simulink model "PFC_69C_03_06_V01_3Phase_3_2KW"  (R2022b)
settings: Solver=FixedStepAuto  StartTime=0.0  StopTime=Inf  RelTol=1e-3  EnableMultiTasking=on
model workspace (MAT data in the model file):
  ADC_Gain = 1241.21212121
  DAC_Gain = 0.000805860805861
  Inductor_Current_Divider_Gain_Phase_A = 33.4
  Inductor_Current_Divider_Gain_Phase_B = 33.4
  Vbulk_Divider_Gain = 276.854928018
  Vin_Divider_Gain = 556.17352614
undefined symbols (not defined in the file or in its folder): GPTRIP1SEL, GPTRIP2SEL, SCI_A_Transmit, SCI_A_Transmit_Current_Suffix, SCI_A_Transmit_one_shot_Suffix, SCI_A_Transmit_Polarity_Suffix, SCI_A_Transmit_relay_Suffix, SCI_A_Transmit_Vbulk_Suffix, SCI_A_Transmit_Vin_rms_Suffix, SCI_A_Transmit_Vin_Suffix, SCI_A_Transmit_Vmid_Suffix, SCI_A_Transmit_Vp_Suffix, SCI_A_Transmit_Vpfc_Suffix, TZ1, TZ2
libraries: c280xlib x38, c2802xlib x34, simulink x17, c2000lib x1
(part 1 of 8)
settings Model: ExtModeTrigDuration=8  Creator=natchammaimuthu  LastModifiedBy=natchammaimuthu
settings OptimizationCC: DefaultUnderspecifiedDataType=single  EnhancedBackFolding=on  PassReuseOutputArgsAs=Individual arguments  MaxStackSize=1024  OptimizeBlockOrder=speed  DifferentSizesBufferReuse=on  OptimizationCustomize=off  DenormalBehavior=FlushToZero  EfficientTunableParamExpr=on
settings DebuggingCC: MultiTaskDSMMsg=none  ParameterPrecisionLossMsg=none  ParameterTunabilityLossMsg=error
settings HardwareCC: ProdBitPerChar=16  ProdBitPerInt=16  ProdBitPerPointer=32  ProdBitPerSizeT=32  ProdBitPerPtrDiffT=32  ProdLargestAtomicInteger=Integer  ProdLargestAtomicFloat=None  ProdWordSize=16  ProdLongLongMode=on  ProdHWDeviceType=Texas Instruments->C2000
settings SFSimCC: MATLABDynamicMemAlloc=off
settings RTWCC: Description=Embedded Coder  SystemTargetFile=ert.tlc  HardwareBoard=TI Piccolo F2806x  TLCOptions=-aInlineSetEventsForThisBaseRateFcn=TLC_FALSE -aSuppressMultiTaskScheduler=TLC_FALSE -aRateBasedStepFcn=1  TemplateMakefile=ert_default_tmf  Toolchain=Texas Instruments Code Composer Studio (C2000)
settings CodeAppCC: ForceParamTrailComments=on  IgnoreCustomStorageClasses=off  OperatorAnnotations=on  SimulinkDataObjDesc=on  SFDataObjDesc=on  InsertBlockDesc=on
settings ERTTargetCC: CodeReplacementLibrary=TI C28x  ExtModeTransport=4  ExtModeStaticAlloc=on  ExtModeAutomaticAllocSize=off  ExtModeMexFile=ext_xcp  ExtModeIntrfLevel=Level2 - Open

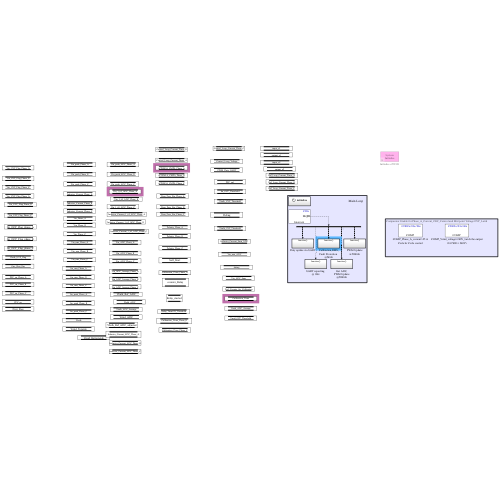
[thumbnail: Simulink's stored preview of the top-level diagram]
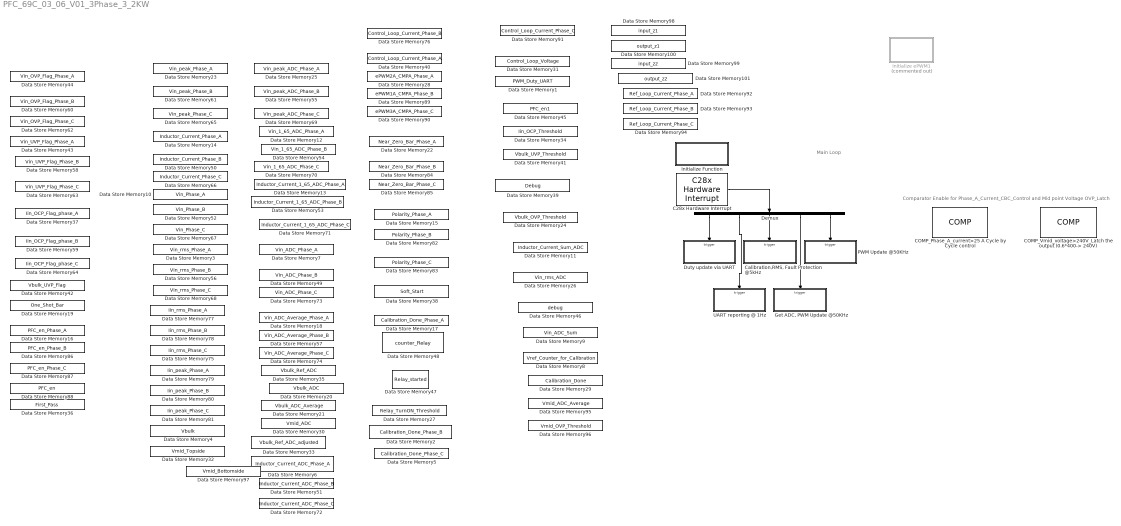
== system PFC_69C_03_06_V01_3Phase_3_2KW ==
  note: Comparator Enable for Phase_A_Current_CBC_Control and Mid point Voltage OVP_Latch
  note: Main Loop
  C28x Hardware Interrupt : c2000lib/Scheduling/C28x Hardware Interrupt  irqnumbers=[9 3 3 3 1]  pienumbers=[1 7 4 2 1]  irqpriorities=[10 9 8 7 6]  irqpreempts=[1 1 1 0 0]  showinput=off  dspchiptype=C280X
  COMP_Phase_A_current>25 A Cycle by Cycle control : c2802xlib/COMP  comparatorModule=Comparator 1  comparatorGPIO1=[]  comparatorGPIO2=0  comparatorSource=Internal DAC  DACOutputValue=744  inverterCircuit=off  synchronizationSelect=Asynchronous  qualificationPeriod=Passed through  Ts=-1
      settings: LibrarySourceBlock=c2806xlib/COMP
  COMP_Vmid_voltage>240V_Latch the output (0.6*400-> 240V) : c2802xlib/COMP  comparatorModule=Comparator 2  comparatorGPIO1=[]  comparatorGPIO2=0  comparatorSource=Internal DAC  DACOutputValue=479  inverterCircuit=off  synchronizationSelect=Asynchronous  qualificationPeriod=Passed through  Ts=-1
      settings: LibrarySourceBlock=c2806xlib/COMP
  "Calibration,RMS, Fault Protection @5kHz" : Subsystem  TreatAsAtomicUnit=on
  Data Store Memory1 : DataStoreMemory  DataStoreName=PWM_Duty_UART  WriteAfterWriteMsg=warning  InitialValue=5  ShowAdditionalParam=off  OutDataTypeStr=double
  Data Store Memory10 : DataStoreMemory  DataStoreName=Vin_Phase_A  WriteAfterWriteMsg=warning  ShowAdditionalParam=off  OutDataTypeStr=double
  Data Store Memory100 : DataStoreMemory  DataStoreName=output_z1  WriteAfterWriteMsg=warning  ShowAdditionalParam=off  OutDataTypeStr=double
  Data Store Memory101 : DataStoreMemory  DataStoreName=output_z2  WriteAfterWriteMsg=warning  ShowAdditionalParam=off  OutDataTypeStr=double
  Data Store Memory11 : DataStoreMemory  DataStoreName=Inductor_Current_Sum_ADC  WriteAfterWriteMsg=warning  ShowAdditionalParam=off  OutDataTypeStr=double
  Data Store Memory12 : DataStoreMemory  DataStoreName=Vin_1_65_ADC_Phase_A  WriteAfterWriteMsg=warning  ShowAdditionalParam=off  OutDataTypeStr=double
  Data Store Memory13 : DataStoreMemory  DataStoreName=Inductor_Current_1_65_ADC_Phase_A  WriteAfterWriteMsg=warning  ShowAdditionalParam=off  OutDataTypeStr=double
  Data Store Memory14 : DataStoreMemory  DataStoreName=Inductor_Current_Phase_A  WriteAfterWriteMsg=warning  ShowAdditionalParam=off  OutDataTypeStr=double
  Data Store Memory15 : DataStoreMemory  DataStoreName=Polarity_Phase_A  WriteAfterWriteMsg=warning  InitialValue=10  ShowAdditionalParam=off
  Data Store Memory16 : DataStoreMemory  DataStoreName=PFC_en_Phase_A  WriteAfterWriteMsg=warning  ShowAdditionalParam=off
  Data Store Memory17 : DataStoreMemory  DataStoreName=Calibration_Done_Phase_A  WriteAfterWriteMsg=warning  ShowAdditionalParam=off  OutDataTypeStr=double
  Data Store Memory18 : DataStoreMemory  DataStoreName=Vin_ADC_Average_Phase_A  WriteAfterWriteMsg=warning  ShowAdditionalParam=off
  Data Store Memory19 : DataStoreMemory  DataStoreName=One_Shot_Bar  WriteAfterWriteMsg=warning  InitialValue=1  ShowAdditionalParam=off  OutDataTypeStr=double
  Data Store Memory2 : DataStoreMemory  DataStoreName=Calibration_Done_Phase_B  WriteAfterWriteMsg=warning  ShowAdditionalParam=off  OutDataTypeStr=double
  Data Store Memory20 : DataStoreMemory  DataStoreName=Vbulk_ADC  WriteAfterWriteMsg=warning  ShowAdditionalParam=off
  Data Store Memory21 : DataStoreMemory  DataStoreName=Vbulk_ADC_Average  WriteAfterWriteMsg=warning  ShowAdditionalParam=off
  Data Store Memory22 : DataStoreMemory  DataStoreName=Near_Zero_Bar_Phase_A  WriteAfterWriteMsg=warning  InitialValue=10  ShowAdditionalParam=off
  Data Store Memory23 : DataStoreMemory  DataStoreName=Vin_peak_Phase_A  WriteAfterWriteMsg=warning  ShowAdditionalParam=off  OutDataTypeStr=double
  Data Store Memory24 : DataStoreMemory  DataStoreName=Vbulk_OVP_Threshold  WriteAfterWriteMsg=warning  InitialValue=100  ShowAdditionalParam=off
  Data Store Memory25 : DataStoreMemory  DataStoreName=Vin_peak_ADC_Phase_A  WriteAfterWriteMsg=warning  ShowAdditionalParam=off  OutDataTypeStr=double
  Data Store Memory26 : DataStoreMemory  DataStoreName=Vin_rms_ADC  WriteAfterWriteMsg=warning  InitialValue=10  ShowAdditionalParam=off
  Data Store Memory27 : DataStoreMemory  DataStoreName=Relay_TurnON_Threshold  WriteAfterWriteMsg=warning  InitialValue=10  ShowAdditionalParam=off
  Data Store Memory28 : DataStoreMemory  DataStoreName=ePWM2A_CMPA_Phase_A  WriteAfterWriteMsg=warning  ShowAdditionalParam=off
  Data Store Memory29 : DataStoreMemory  DataStoreName=Calibration_Done  WriteAfterWriteMsg=warning  ShowAdditionalParam=off  OutDataTypeStr=double
  Data Store Memory3 : DataStoreMemory  DataStoreName=Vin_rms_Phase_A  WriteAfterWriteMsg=warning  InitialValue=10  ShowAdditionalParam=off
  Data Store Memory30 : DataStoreMemory  DataStoreName=Vmid_ADC  WriteAfterWriteMsg=warning  InitialValue=10  ShowAdditionalParam=off  OutDataTypeStr=double
  Data Store Memory31 : DataStoreMemory  DataStoreName=Control_Loop_Voltage  WriteAfterWriteMsg=warning  InitialValue=100  ShowAdditionalParam=off
  Data Store Memory32 : DataStoreMemory  DataStoreName=Vmid_Topside  WriteAfterWriteMsg=warning  InitialValue=10  ShowAdditionalParam=off  OutDataTypeStr=double
  Data Store Memory33 : DataStoreMemory  DataStoreName=Vbulk_Ref_ADC_adjusted  WriteAfterWriteMsg=warning  InitialValue=10  ShowAdditionalParam=off  OutDataTypeStr=double
  Data Store Memory34 : DataStoreMemory  DataStoreName=Iin_OCP_Threshold  WriteAfterWriteMsg=warning  ShowAdditionalParam=off  OutDataTypeStr=double
  Data Store Memory35 : DataStoreMemory  DataStoreName=Vbulk_Ref_ADC  WriteAfterWriteMsg=warning  InitialValue=10  ShowAdditionalParam=off  OutDataTypeStr=double
  Data Store Memory36 : DataStoreMemory  DataStoreName=First_Pass  WriteAfterWriteMsg=warning  ShowAdditionalParam=off  OutDataTypeStr=double
  Data Store Memory37 : DataStoreMemory  DataStoreName=Iin_OCP_Flag_phase_A  WriteAfterWriteMsg=warning  InitialValue=1  ShowAdditionalParam=off  OutDataTypeStr=double
  Data Store Memory38 : DataStoreMemory  DataStoreName=Soft_Start  WriteAfterWriteMsg=warning  InitialValue=10  ShowAdditionalParam=off  OutDataTypeStr=double
  Data Store Memory39 : DataStoreMemory  DataStoreName=Debug  WriteAfterWriteMsg=warning  InitialValue=10  ShowAdditionalParam=off  OutDataTypeStr=double
  Data Store Memory4 : DataStoreMemory  DataStoreName=Vbulk  WriteAfterWriteMsg=warning  ShowAdditionalParam=off  OutDataTypeStr=double
  Data Store Memory40 : DataStoreMemory  DataStoreName=Control_Loop_Current_Phase_A  WriteAfterWriteMsg=warning  InitialValue=100  ShowAdditionalParam=off
  Data Store Memory41 : DataStoreMemory  DataStoreName=Vbulk_UVP_Threshold  WriteAfterWriteMsg=warning  InitialValue=-10  VectorParams1D=off  ShowAdditionalParam=off  OutDataTypeStr=double
  Data Store Memory42 : DataStoreMemory  DataStoreName=Vbulk_UVP_Flag  WriteAfterWriteMsg=warning  ShowAdditionalParam=off
  Data Store Memory43 : DataStoreMemory  DataStoreName=Vin_UVP_Flag_Phase_A  WriteAfterWriteMsg=warning  ShowAdditionalParam=off
  Data Store Memory44 : DataStoreMemory  DataStoreName=Vin_OVP_Flag_Phase_A  WriteAfterWriteMsg=warning  ShowAdditionalParam=off
  Data Store Memory45 : DataStoreMemory  DataStoreName=PFC_en1  WriteAfterWriteMsg=warning  ShowAdditionalParam=off
  Data Store Memory46 : DataStoreMemory  DataStoreName=debug  WriteAfterWriteMsg=warning  ShowAdditionalParam=off
  Data Store Memory47 : DataStoreMemory  DataStoreName=Relay_started  WriteAfterWriteMsg=warning  ShowAdditionalParam=off
  Data Store Memory48 : DataStoreMemory  DataStoreName=counter_Relay  WriteAfterWriteMsg=warning  ShowAdditionalParam=off
  Data Store Memory49 : DataStoreMemory  DataStoreName=Vin_ADC_Phase_B  WriteAfterWriteMsg=warning  ShowAdditionalParam=off
  Data Store Memory5 : DataStoreMemory  DataStoreName=Calibration_Done_Phase_C  WriteAfterWriteMsg=warning  ShowAdditionalParam=off  OutDataTypeStr=double
  Data Store Memory50 : DataStoreMemory  DataStoreName=Inductor_Current_Phase_B  WriteAfterWriteMsg=warning  ShowAdditionalParam=off  OutDataTypeStr=double
  Data Store Memory51 : DataStoreMemory  DataStoreName=Inductor_Current_ADC_Phase_B  WriteAfterWriteMsg=warning  ShowAdditionalParam=off  OutDataTypeStr=double
  Data Store Memory52 : DataStoreMemory  DataStoreName=Vin_Phase_B  WriteAfterWriteMsg=warning  ShowAdditionalParam=off  OutDataTypeStr=double
  Data Store Memory53 : DataStoreMemory  DataStoreName=Inductor_Current_1_65_ADC_Phase_B  WriteAfterWriteMsg=warning  ShowAdditionalParam=off  OutDataTypeStr=double
  Data Store Memory54 : DataStoreMemory  DataStoreName=Vin_1_65_ADC_Phase_B  WriteAfterWriteMsg=warning  ShowAdditionalParam=off  OutDataTypeStr=double
  Data Store Memory55 : DataStoreMemory  DataStoreName=Vin_peak_ADC_Phase_B  WriteAfterWriteMsg=warning  ShowAdditionalParam=off  OutDataTypeStr=double
  Data Store Memory56 : DataStoreMemory  DataStoreName=Vin_rms_Phase_B  WriteAfterWriteMsg=warning  InitialValue=10  ShowAdditionalParam=off
  Data Store Memory57 : DataStoreMemory  DataStoreName=Vin_ADC_Average_Phase_B  WriteAfterWriteMsg=warning  ShowAdditionalParam=off
  Data Store Memory58 : DataStoreMemory  DataStoreName=Vin_UVP_Flag_Phase_B  WriteAfterWriteMsg=warning  ShowAdditionalParam=off
  Data Store Memory59 : DataStoreMemory  DataStoreName=Iin_OCP_Flag_phase_B  WriteAfterWriteMsg=warning  InitialValue=1  ShowAdditionalParam=off  OutDataTypeStr=double
  Data Store Memory6 : DataStoreMemory  DataStoreName=Inductor_Current_ADC_Phase_A  WriteAfterWriteMsg=warning  ShowAdditionalParam=off  OutDataTypeStr=double
  Data Store Memory60 : DataStoreMemory  DataStoreName=Vin_OVP_Flag_Phase_B  WriteAfterWriteMsg=warning  ShowAdditionalParam=off
  Data Store Memory61 : DataStoreMemory  DataStoreName=Vin_peak_Phase_B  WriteAfterWriteMsg=warning  ShowAdditionalParam=off  OutDataTypeStr=double
  Data Store Memory62 : DataStoreMemory  DataStoreName=Vin_OVP_Flag_Phase_C  WriteAfterWriteMsg=warning  ShowAdditionalParam=off
  Data Store Memory63 : DataStoreMemory  DataStoreName=Vin_UVP_Flag_Phase_C  WriteAfterWriteMsg=warning  ShowAdditionalParam=off
  Data Store Memory64 : DataStoreMemory  DataStoreName=Iin_OCP_Flag_phase_C  WriteAfterWriteMsg=warning  InitialValue=1  ShowAdditionalParam=off  OutDataTypeStr=double
  Data Store Memory65 : DataStoreMemory  DataStoreName=Vin_peak_Phase_C  WriteAfterWriteMsg=warning  ShowAdditionalParam=off  OutDataTypeStr=double
  Data Store Memory66 : DataStoreMemory  DataStoreName=Inductor_Current_Phase_C  WriteAfterWriteMsg=warning  ShowAdditionalParam=off  OutDataTypeStr=double
  Data Store Memory67 : DataStoreMemory  DataStoreName=Vin_Phase_C  WriteAfterWriteMsg=warning  ShowAdditionalParam=off  OutDataTypeStr=double
  Data Store Memory68 : DataStoreMemory  DataStoreName=Vin_rms_Phase_C  WriteAfterWriteMsg=warning  InitialValue=10  ShowAdditionalParam=off
  Data Store Memory69 : DataStoreMemory  DataStoreName=Vin_peak_ADC_Phase_C  WriteAfterWriteMsg=warning  ShowAdditionalParam=off  OutDataTypeStr=double
  Data Store Memory7 : DataStoreMemory  DataStoreName=Vin_ADC_Phase_A  WriteAfterWriteMsg=warning  ShowAdditionalParam=off
  Data Store Memory70 : DataStoreMemory  DataStoreName=Vin_1_65_ADC_Phase_C  WriteAfterWriteMsg=warning  ShowAdditionalParam=off  OutDataTypeStr=double
  Data Store Memory71 : DataStoreMemory  DataStoreName=Inductor_Current_1_65_ADC_Phase_C  WriteAfterWriteMsg=warning  ShowAdditionalParam=off  OutDataTypeStr=double
  Data Store Memory72 : DataStoreMemory  DataStoreName=Inductor_Current_ADC_Phase_C  WriteAfterWriteMsg=warning  ShowAdditionalParam=off  OutDataTypeStr=double
  Data Store Memory73 : DataStoreMemory  DataStoreName=Vin_ADC_Phase_C  WriteAfterWriteMsg=warning  ShowAdditionalParam=off
  Data Store Memory74 : DataStoreMemory  DataStoreName=Vin_ADC_Average_Phase_C  WriteAfterWriteMsg=warning  ShowAdditionalParam=off
  Data Store Memory75 : DataStoreMemory  DataStoreName=Iin_rms_Phase_C  WriteAfterWriteMsg=warning  InitialValue=10  ShowAdditionalParam=off
  Data Store Memory76 : DataStoreMemory  DataStoreName=Control_Loop_Current_Phase_B  WriteAfterWriteMsg=warning  InitialValue=100  ShowAdditionalParam=off
  Data Store Memory77 : DataStoreMemory  DataStoreName=Iin_rms_Phase_A  WriteAfterWriteMsg=warning  InitialValue=10  ShowAdditionalParam=off
  Data Store Memory78 : DataStoreMemory  DataStoreName=Iin_rms_Phase_B  WriteAfterWriteMsg=warning  InitialValue=10  ShowAdditionalParam=off
  Data Store Memory79 : DataStoreMemory  DataStoreName=Iin_peak_Phase_A  WriteAfterWriteMsg=warning  ShowAdditionalParam=off  OutDataTypeStr=double
  Data Store Memory8 : DataStoreMemory  DataStoreName=Vref_Counter_for_Calibration  WriteAfterWriteMsg=warning  ShowAdditionalParam=off
  Data Store Memory80 : DataStoreMemory  DataStoreName=Iin_peak_Phase_B  WriteAfterWriteMsg=warning  ShowAdditionalParam=off  OutDataTypeStr=double
  Data Store Memory81 : DataStoreMemory  DataStoreName=Iin_peak_Phase_C  WriteAfterWriteMsg=warning  ShowAdditionalParam=off  OutDataTypeStr=double
  Data Store Memory82 : DataStoreMemory  DataStoreName=Polarity_Phase_B  WriteAfterWriteMsg=warning  InitialValue=10  ShowAdditionalParam=off
  Data Store Memory83 : DataStoreMemory  DataStoreName=Polarity_Phase_C  WriteAfterWriteMsg=warning  InitialValue=10  ShowAdditionalParam=off
  Data Store Memory84 : DataStoreMemory  DataStoreName=Near_Zero_Bar_Phase_B  WriteAfterWriteMsg=warning  InitialValue=10  ShowAdditionalParam=off
  Data Store Memory85 : DataStoreMemory  DataStoreName=Near_Zero_Bar_Phase_C  WriteAfterWriteMsg=warning  InitialValue=10  ShowAdditionalParam=off
  Data Store Memory86 : DataStoreMemory  DataStoreName=PFC_en_Phase_B  WriteAfterWriteMsg=warning  ShowAdditionalParam=off
  Data Store Memory87 : DataStoreMemory  DataStoreName=PFC_en_Phase_C  WriteAfterWriteMsg=warning  ShowAdditionalParam=off
  Data Store Memory88 : DataStoreMemory  DataStoreName=PFC_en  WriteAfterWriteMsg=warning  ShowAdditionalParam=off
  Data Store Memory89 : DataStoreMemory  DataStoreName=ePWM1A_CMPA_Phase_B  WriteAfterWriteMsg=warning  ShowAdditionalParam=off
  Data Store Memory9 : DataStoreMemory  DataStoreName=Vin_ADC_Sum  WriteAfterWriteMsg=warning  ShowAdditionalParam=off  OutDataTypeStr=double
  Data Store Memory90 : DataStoreMemory  DataStoreName=ePWM3A_CMPA_Phase_C  WriteAfterWriteMsg=warning  ShowAdditionalParam=off
  Data Store Memory91 : DataStoreMemory  DataStoreName=Control_Loop_Current_Phase_C  WriteAfterWriteMsg=warning  InitialValue=100  ShowAdditionalParam=off
  Data Store Memory92 : DataStoreMemory  DataStoreName=Ref_Loop_Current_Phase_A  WriteAfterWriteMsg=warning  InitialValue=100  ShowAdditionalParam=off
  Data Store Memory93 : DataStoreMemory  DataStoreName=Ref_Loop_Current_Phase_B  WriteAfterWriteMsg=warning  InitialValue=100  ShowAdditionalParam=off
  Data Store Memory94 : DataStoreMemory  DataStoreName=Ref_Loop_Current_Phase_C  WriteAfterWriteMsg=warning  InitialValue=100  ShowAdditionalParam=off
  Data Store Memory95 : DataStoreMemory  DataStoreName=Vmid_ADC_Average  WriteAfterWriteMsg=warning  ShowAdditionalParam=off
  Data Store Memory96 : DataStoreMemory  DataStoreName=Vmid_OVP_Threshold  WriteAfterWriteMsg=warning  InitialValue=100  ShowAdditionalParam=off
  Data Store Memory97 : DataStoreMemory  DataStoreName=Vmid_Bottomside  WriteAfterWriteMsg=warning  InitialValue=10  ShowAdditionalParam=off  OutDataTypeStr=double
  Data Store Memory98 : DataStoreMemory  DataStoreName=input_z1  WriteAfterWriteMsg=warning  ShowAdditionalParam=off  OutDataTypeStr=double
  Data Store Memory99 : DataStoreMemory  DataStoreName=input_z2  WriteAfterWriteMsg=warning  ShowAdditionalParam=off  OutDataTypeStr=double
  Demux : Demux  Outputs=5
  Duty update via UART : Subsystem  TreatAsAtomicUnit=on
  "Get ADC, PWM Update @50KHz" : Subsystem  TreatAsAtomicUnit=on
  Initialize Function : Subsystem  TreatAsAtomicUnit=on
  Initialize ePWM1 : Subsystem  Commented=on  mask(System Initialize){ShowInLibBrowser=0}
      mask prompts: ShowInLibBrowser "Simulink:masks:CustCodeMaskParam1_MP"
      settings: CopyFcn=cccopyfcn(gcb)  OpenFcn=ccopenfcn('System Initialize Function')
      mask Help: eval('feval(''rtwprivate'',''rtwhelpview'',''rtw_sys_initialize_block'')');
      mask Display: disp('System\nInitialize');
  PWM Update @50KHz : Subsystem  TreatAsAtomicUnit=on
  UART reporting @ 1Hz : Subsystem  TreatAsAtomicUnit=on
  wires:
  C28x Hardware Interrupt/1 -> Demux/1
  Demux/1 -> Duty update via UART/Trigger
  Demux/4 -> "Get ADC, PWM Update @50KHz"/Trigger
  Demux/5 -> PWM Update @50KHz/Trigger
  Demux/3 -> "Calibration,RMS, Fault Protection @5kHz"/Trigger
  Demux/2 -> UART reporting @ 1Hz/Trigger

== system PFC_69C_03_06_V01_3Phase_3_2KW/Calibration,RMS, Fault Protection @5kHz ==
  function : TriggerPort  TriggerType=function-call  VariantControl=(inherit)
  Calibration : Subsystem  TreatAsAtomicUnit=on
  Current_Control_REF_Adjusted_Phase_A : Subsystem  TreatAsAtomicUnit=on
  Current_Control_REF_Adjusted_Phase_B : Subsystem  TreatAsAtomicUnit=on
  Current_Control_REF_Adjusted_Phase_C : Subsystem  TreatAsAtomicUnit=on
  Fault checking : Subsystem  TreatAsAtomicUnit=on
  Function-Call Generator : simulink/Ports & Subsystems/Function-Call Generator  sample_time=-1  numberOfIterations=1  DisallowWideOutput=off
  Function-Call Split : FunctionCallSplit  IconShape=distinctive  NumOutputPorts=12  OutputPortLayout=default
  PFC_en and output/input : Subsystem  TreatAsAtomicUnit=on
  Polarity & Near Zero check : Subsystem  TreatAsAtomicUnit=on
  Relay control : Subsystem  Commented=on  TreatAsAtomicUnit=on
  Relay control_corrected : Subsystem  TreatAsAtomicUnit=on
  Soft Start : Subsystem  TreatAsAtomicUnit=on
  Voltage RMS/Averag Calculation : Subsystem  TreatAsAtomicUnit=on
  Voltage loop PWM generation (Control) : Subsystem  TreatAsAtomicUnit=on
  Voltage sensing : Subsystem  Commented=on  TreatAsAtomicUnit=on
  wires:
  Function-Call Generator/1 -> Function-Call Split/1
  Function-Call Split/12 -> Current_Control_REF_Adjusted_Phase_C/Trigger
  Function-Call Split/11 -> Current_Control_REF_Adjusted_Phase_B/Trigger
  Function-Call Split/10 -> Current_Control_REF_Adjusted_Phase_A/Trigger
  Function-Call Split/9 -> Voltage loop PWM generation (Control)/Trigger
  Function-Call Split/8 -> PFC_en and output/input/Trigger
  Function-Call Split/7 -> Soft Start/Trigger
  Function-Call Split/6 -> Relay control_corrected/Trigger
  Function-Call Split/5 -> Polarity & Near Zero check/Trigger
  Function-Call Split/4 -> Fault checking/Trigger
  Function-Call Split/3 -> Voltage RMS/Averag Calculation/Trigger
  Function-Call Split/2 -> Calibration/Trigger
  Function-Call Split/1 -> Voltage sensing/Trigger

== system PFC_69C_03_06_V01_3Phase_3_2KW/Duty update via UART ==
  function : TriggerPort  TriggerType=function-call  VariantControl=(inherit)
  Data Store Write1 : DataStoreWrite  DataStoreName=PWM_Duty_UART  IndexOptions=Index vector (dialog)  Indices=1  OutputSizes=1
  Function Caller : FunctionCaller  FunctionPrototype=y = SCI_Receive()  InputArgumentSpecifications=<Enter example>  OutputArgumentSpecifications=<Enter example>
  Simulink Function : Subsystem  TreatAsAtomicUnit=on
  wires:
  Function Caller/1 -> Data Store Write1/1

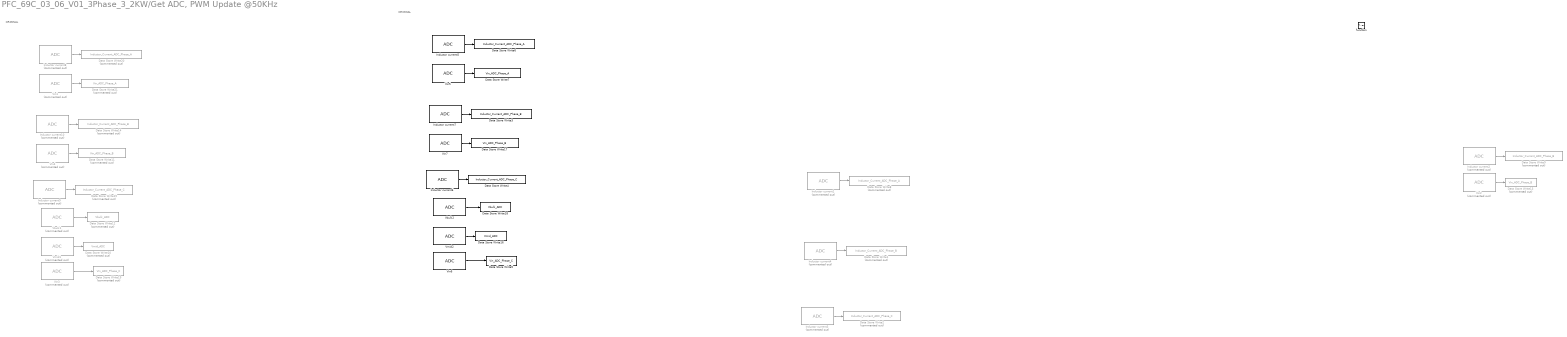
== system PFC_69C_03_06_V01_3Phase_3_2KW/Get ADC, PWM Update @50KHz ==
  note: ORIGINAL
  note: ORIGINAL
  function : TriggerPort  TriggerType=function-call  VariantControl=(inherit)
  Data Store Write1 : DataStoreWrite  Commented=on  DataStoreName=Inductor_Current_ADC_Phase_B  IndexOptions=Index vector (dialog)  Indices=1  OutputSizes=1
  Data Store Write10 : DataStoreWrite  Commented=on  DataStoreName=Vmid_ADC  IndexOptions=Index vector (dialog)  Indices=1  OutputSizes=1
  Data Store Write11 : DataStoreWrite  Commented=on  DataStoreName=Vin_ADC_Phase_B  IndexOptions=Index vector (dialog)  Indices=1  OutputSizes=1
  Data Store Write12 : DataStoreWrite  Commented=on  DataStoreName=Vbulk_ADC  IndexOptions=Index vector (dialog)  Indices=1  OutputSizes=1
  Data Store Write13 : DataStoreWrite  Commented=on  DataStoreName=Vin_ADC_Phase_B  IndexOptions=Index vector (dialog)  Indices=1  OutputSizes=1
  Data Store Write14 : DataStoreWrite  Commented=on  DataStoreName=Inductor_Current_ADC_Phase_B  IndexOptions=Index vector (dialog)  Indices=1  OutputSizes=1
  Data Store Write15 : DataStoreWrite  Commented=on  DataStoreName=Inductor_Current_ADC_Phase_C  IndexOptions=Index vector (dialog)  Indices=1  OutputSizes=1
  Data Store Write16 : DataStoreWrite  DataStoreName=Vmid_ADC  IndexOptions=Index vector (dialog)  Indices=1  OutputSizes=1
  Data Store Write17 : DataStoreWrite  DataStoreName=Vin_ADC_Phase_B  IndexOptions=Index vector (dialog)  Indices=1  OutputSizes=1
  Data Store Write18 : DataStoreWrite  DataStoreName=Vbulk_ADC  IndexOptions=Index vector (dialog)  Indices=1  OutputSizes=1
  Data Store Write19 : DataStoreWrite  Commented=on  DataStoreName=Vin_ADC_Phase_C  IndexOptions=Index vector (dialog)  Indices=1  OutputSizes=1
  Data Store Write2 : DataStoreWrite  Commented=on  DataStoreName=Inductor_Current_ADC_Phase_C  IndexOptions=Index vector (dialog)  Indices=1  OutputSizes=1
  Data Store Write20 : DataStoreWrite  Commented=on  DataStoreName=Inductor_Current_ADC_Phase_A  IndexOptions=Index vector (dialog)  Indices=1  OutputSizes=1
  Data Store Write21 : DataStoreWrite  Commented=on  DataStoreName=Vin_ADC_Phase_A  IndexOptions=Index vector (dialog)  Indices=1  OutputSizes=1
  Data Store Write3 : DataStoreWrite  DataStoreName=Inductor_Current_ADC_Phase_B  IndexOptions=Index vector (dialog)  Indices=1  OutputSizes=1
  Data Store Write4 : DataStoreWrite  DataStoreName=Inductor_Current_ADC_Phase_C  IndexOptions=Index vector (dialog)  Indices=1  OutputSizes=1
  Data Store Write5 : DataStoreWrite  DataStoreName=Vin_ADC_Phase_C  IndexOptions=Index vector (dialog)  Indices=1  OutputSizes=1
  Data Store Write6 : DataStoreWrite  DataStoreName=Inductor_Current_ADC_Phase_A  IndexOptions=Index vector (dialog)  Indices=1  OutputSizes=1
  Data Store Write7 : DataStoreWrite  DataStoreName=Vin_ADC_Phase_A  IndexOptions=Index vector (dialog)  Indices=1  OutputSizes=1
  Data Store Write8 : DataStoreWrite  Commented=on  DataStoreName=Inductor_Current_ADC_Phase_A  IndexOptions=Index vector (dialog)  Indices=1  OutputSizes=1
  Data Store Write9 : DataStoreWrite  Commented=on  DataStoreName=Inductor_Current_ADC_Phase_B  IndexOptions=Index vector (dialog)  Indices=1  OutputSizes=1
  Inductor current1 : c2802xlib/ADC  Commented=on  blkParamProc=C2000  ADCModule=1  samplingMode=Single sample mode  ADCResolution=12-bit (Single-ended input)  useSOC1=SOC0  useSOC2=SOC0_SOC1  SOCAcquisitionWindow=7  SOCTriggerSource=Software  SOCInterruptTrigger=No ADCINT  Ts=-1  dType=double  postInterrupt=off  interruptSel=ADCINT1  ADCINTContinuous=off  endma=off  chdma=1  conv1=ADCINA2  conv2=ADCINA0 and ADCINB0  conv1_Type4=ADCIN0  conv2_Type4=ADCIN0 and ADCIN1
      settings: LibrarySourceBlock=c2806xlib/ADC
  Inductor current10 : c2802xlib/ADC  Commented=on  blkParamProc=C2000  ADCModule=1  samplingMode=Single sample mode  ADCResolution=12-bit (Single-ended input)  useSOC1=SOC1  useSOC2=SOC0_SOC1  SOCAcquisitionWindow=10  SOCTriggerSource=ePWM2_ADCSOCA  SOCInterruptTrigger=No ADCINT  Ts=-1  dType=double  postInterrupt=off  interruptSel=ADCINT1  ADCINTContinuous=off  endma=off  chdma=1  conv1=ADCINA1  conv2=ADCINA0 and ADCINB0  conv1_Type4=ADCIN0  conv2_Type4=ADCIN0 and ADCIN1
      settings: LibrarySourceBlock=c2806xlib/ADC
  Inductor current2 : c2802xlib/ADC  Commented=on  blkParamProc=C2000  ADCModule=1  samplingMode=Single sample mode  ADCResolution=12-bit (Single-ended input)  useSOC1=SOC0  useSOC2=SOC0_SOC1  SOCAcquisitionWindow=10  SOCTriggerSource=ePWM1_ADCSOCA  SOCInterruptTrigger=No ADCINT  Ts=-1  dType=double  postInterrupt=off  interruptSel=ADCINT1  ADCINTContinuous=off  endma=off  chdma=1  conv1=ADCINA1  conv2=ADCINA0 and ADCINB0  conv1_Type4=ADCIN0  conv2_Type4=ADCIN0 and ADCIN1
      settings: LibrarySourceBlock=c2806xlib/ADC
  Inductor current3 : c2802xlib/ADC  Commented=on  blkParamProc=C2000  ADCModule=1  samplingMode=Single sample mode  ADCResolution=12-bit (Single-ended input)  useSOC1=SOC2  useSOC2=SOC4_SOC5  SOCAcquisitionWindow=7  SOCTriggerSource=Software  SOCInterruptTrigger=No ADCINT  Ts=-1  dType=double  postInterrupt=on  interruptSel=ADCINT1  ADCINTContinuous=on  endma=off  chdma=1  conv1=ADCINA0  conv2=ADCINA0 and ADCINB0  conv1_Type4=ADCIN0  conv2_Type4=ADCIN0 and ADCIN1
      settings: LibrarySourceBlock=c2806xlib/ADC
  Inductor current4 : c2802xlib/ADC  Commented=on  blkParamProc=C2000  ADCModule=1  samplingMode=Single sample mode  ADCResolution=12-bit (Single-ended input)  useSOC1=SOC1  useSOC2=SOC0_SOC1  SOCAcquisitionWindow=7  SOCTriggerSource=Software  SOCInterruptTrigger=No ADCINT  Ts=-1  dType=double  postInterrupt=off  interruptSel=ADCINT1  ADCINTContinuous=off  endma=off  chdma=1  conv1=ADCINA1  conv2=ADCINA0 and ADCINB0  conv1_Type4=ADCIN0  conv2_Type4=ADCIN0 and ADCIN1
      settings: LibrarySourceBlock=c2806xlib/ADC
  Inductor current5 : c2802xlib/ADC  blkParamProc=C2000  ADCModule=1  samplingMode=Single sample mode  ADCResolution=12-bit (Single-ended input)  useSOC1=SOC4  useSOC2=SOC0_SOC1  SOCAcquisitionWindow=7  SOCTriggerSource=ePWM2_ADCSOCA  SOCInterruptTrigger=No ADCINT  Ts=-1  dType=double  postInterrupt=off  interruptSel=ADCINT1  ADCINTContinuous=off  endma=off  chdma=1  conv1=ADCINA2  conv2=ADCINA0 and ADCINB0  conv1_Type4=ADCIN0  conv2_Type4=ADCIN0 and ADCIN1
      settings: LibrarySourceBlock=c2806xlib/ADC
  Inductor current6 : c2802xlib/ADC  blkParamProc=C2000  ADCModule=1  samplingMode=Single sample mode  ADCResolution=12-bit (Single-ended input)  useSOC1=SOC6  useSOC2=SOC4_SOC5  SOCAcquisitionWindow=7  SOCTriggerSource=ePWM2_ADCSOCA  SOCInterruptTrigger=No ADCINT  Ts=-1  dType=double  postInterrupt=off  interruptSel=ADCINT1  ADCINTContinuous=off  endma=off  chdma=1  conv1=ADCINA0  conv2=ADCINA0 and ADCINB0  conv1_Type4=ADCIN0  conv2_Type4=ADCIN0 and ADCIN1
      settings: LibrarySourceBlock=c2806xlib/ADC
  Inductor current7 : c2802xlib/ADC  blkParamProc=C2000  ADCModule=1  samplingMode=Single sample mode  ADCResolution=12-bit (Single-ended input)  useSOC1=SOC1  useSOC2=SOC0_SOC1  SOCAcquisitionWindow=7  SOCTriggerSource=ePWM2_ADCSOCA  SOCInterruptTrigger=No ADCINT  Ts=-1  dType=double  postInterrupt=off  interruptSel=ADCINT1  ADCINTContinuous=off  endma=off  chdma=1  conv1=ADCINA1  conv2=ADCINA0 and ADCINB0  conv1_Type4=ADCIN0  conv2_Type4=ADCIN0 and ADCIN1
      settings: LibrarySourceBlock=c2806xlib/ADC
  Inductor current8 : c2802xlib/ADC  Commented=on  blkParamProc=C2000  ADCModule=1  samplingMode=Single sample mode  ADCResolution=12-bit (Single-ended input)  useSOC1=SOC4  useSOC2=SOC0_SOC1  SOCAcquisitionWindow=10  SOCTriggerSource=ePWM2_ADCSOCA  SOCInterruptTrigger=No ADCINT  Ts=-1  dType=double  postInterrupt=off  interruptSel=ADCINT1  ADCINTContinuous=off  endma=off  chdma=1  conv1=ADCINA2  conv2=ADCINA0 and ADCINB0  conv1_Type4=ADCIN0  conv2_Type4=ADCIN0 and ADCIN1
      settings: LibrarySourceBlock=c2806xlib/ADC
  Inductor current9 : c2802xlib/ADC  Commented=on  blkParamProc=C2000  ADCModule=1  samplingMode=Single sample mode  ADCResolution=12-bit (Single-ended input)  useSOC1=SOC6  useSOC2=SOC4_SOC5  SOCAcquisitionWindow=10  SOCTriggerSource=ePWM2_ADCSOCA  SOCInterruptTrigger=No ADCINT  Ts=-1  dType=double  postInterrupt=off  interruptSel=ADCINT1  ADCINTContinuous=off  endma=off  chdma=1  conv1=ADCINA0  conv2=ADCINA0 and ADCINB0  conv1_Type4=ADCIN0  conv2_Type4=ADCIN0 and ADCIN1
      settings: LibrarySourceBlock=c2806xlib/ADC
  Vbulk1 : c2802xlib/ADC  Commented=on  blkParamProc=C2000  ADCModule=1  samplingMode=Single sample mode  ADCResolution=12-bit (Single-ended input)  useSOC1=SOC0  useSOC2=SOC0_SOC1  SOCAcquisitionWindow=10  SOCTriggerSource=ePWM2_ADCSOCA  SOCInterruptTrigger=No ADCINT  Ts=-1  dType=double  postInterrupt=off  interruptSel=ADCINT1  ADCINTContinuous=off  endma=off  chdma=1  conv1=ADCINA3  conv2=ADCINA0 and ADCINB0  conv1_Type4=ADCIN0  conv2_Type4=ADCIN0 and ADCIN1
      settings: LibrarySourceBlock=c2806xlib/ADC
  Vbulk2 : c2802xlib/ADC  blkParamProc=C2000  ADCModule=1  samplingMode=Single sample mode  ADCResolution=12-bit (Single-ended input)  useSOC1=SOC0  useSOC2=SOC0_SOC1  SOCAcquisitionWindow=7  SOCTriggerSource=ePWM2_ADCSOCA  SOCInterruptTrigger=No ADCINT  Ts=-1  dType=double  postInterrupt=off  interruptSel=ADCINT1  ADCINTContinuous=off  endma=off  chdma=1  conv1=ADCINA3  conv2=ADCINA0 and ADCINB0  conv1_Type4=ADCIN0  conv2_Type4=ADCIN0 and ADCIN1
      settings: LibrarySourceBlock=c2806xlib/ADC
  Vin1 : c2802xlib/ADC  Commented=on  blkParamProc=C2000  ADCModule=1  samplingMode=Single sample mode  ADCResolution=12-bit (Single-ended input)  useSOC1=SOC5  useSOC2=SOC2_SOC3  SOCAcquisitionWindow=10  SOCTriggerSource=ePWM2_ADCSOCA  SOCInterruptTrigger=No ADCINT  Ts=-1  dType=double  postInterrupt=off  interruptSel=ADCINT1  ADCINTContinuous=off  endma=off  chdma=1  conv1=ADCINB2  conv2=ADCINA0 and ADCINB0  conv1_Type4=ADCIN0  conv2_Type4=ADCIN0 and ADCIN1
      settings: LibrarySourceBlock=c2806xlib/ADC
  Vin2 : c2802xlib/ADC  Commented=on  blkParamProc=C2000  ADCModule=1  samplingMode=Single sample mode  ADCResolution=12-bit (Single-ended input)  useSOC1=SOC1  useSOC2=SOC0_SOC1  SOCAcquisitionWindow=10  SOCTriggerSource=ePWM1_ADCSOCA  SOCInterruptTrigger=No ADCINT  Ts=-1  dType=double  postInterrupt=off  interruptSel=ADCINT1  ADCINTContinuous=off  endma=off  chdma=1  conv1=ADCINB1  conv2=ADCINA0 and ADCINB0  conv1_Type4=ADCIN0  conv2_Type4=ADCIN0 and ADCIN1
      settings: LibrarySourceBlock=c2806xlib/ADC
  Vin3 : c2802xlib/ADC  Commented=on  blkParamProc=C2000  ADCModule=1  samplingMode=Single sample mode  ADCResolution=12-bit (Single-ended input)  useSOC1=SOC7  useSOC2=SOC6_SOC7  SOCAcquisitionWindow=10  SOCTriggerSource=ePWM2_ADCSOCA  SOCInterruptTrigger=No ADCINT  Ts=-1  dType=double  postInterrupt=on  interruptSel=ADCINT1  ADCINTContinuous=on  endma=off  chdma=1  conv1=ADCINB0  conv2=ADCINA0 and ADCINB0  conv1_Type4=ADCIN0  conv2_Type4=ADCIN0 and ADCIN1
      settings: LibrarySourceBlock=c2806xlib/ADC
  Vin4 : c2802xlib/ADC  Commented=on  blkParamProc=C2000  ADCModule=1  samplingMode=Single sample mode  ADCResolution=12-bit (Single-ended input)  useSOC1=SOC2  useSOC2=SOC2_SOC3  SOCAcquisitionWindow=10  SOCTriggerSource=ePWM2_ADCSOCA  SOCInterruptTrigger=No ADCINT  Ts=-1  dType=double  postInterrupt=off  interruptSel=ADCINT1  ADCINTContinuous=off  endma=off  chdma=1  conv1=ADCINB1  conv2=ADCINA0 and ADCINB0  conv1_Type4=ADCIN0  conv2_Type4=ADCIN0 and ADCIN1
      settings: LibrarySourceBlock=c2806xlib/ADC
  Vin5 : c2802xlib/ADC  blkParamProc=C2000  ADCModule=1  samplingMode=Single sample mode  ADCResolution=12-bit (Single-ended input)  useSOC1=SOC5  useSOC2=SOC2_SOC3  SOCAcquisitionWindow=7  SOCTriggerSource=ePWM2_ADCSOCA  SOCInterruptTrigger=No ADCINT  Ts=-1  dType=double  postInterrupt=off  interruptSel=ADCINT1  ADCINTContinuous=off  endma=off  chdma=1  conv1=ADCINB2  conv2=ADCINA0 and ADCINB0  conv1_Type4=ADCIN0  conv2_Type4=ADCIN0 and ADCIN1
      settings: LibrarySourceBlock=c2806xlib/ADC
  Vin6 : c2802xlib/ADC  blkParamProc=C2000  ADCModule=1  samplingMode=Single sample mode  ADCResolution=12-bit (Single-ended input)  useSOC1=SOC7  useSOC2=SOC6_SOC7  SOCAcquisitionWindow=7  SOCTriggerSource=ePWM2_ADCSOCA  SOCInterruptTrigger=No ADCINT  Ts=-1  dType=double  postInterrupt=on  interruptSel=ADCINT1  ADCINTContinuous=on  endma=off  chdma=1  conv1=ADCINB0  conv2=ADCINA0 and ADCINB0  conv1_Type4=ADCIN0  conv2_Type4=ADCIN0 and ADCIN1
      settings: LibrarySourceBlock=c2806xlib/ADC
  Vin7 : c2802xlib/ADC  blkParamProc=C2000  ADCModule=1  samplingMode=Single sample mode  ADCResolution=12-bit (Single-ended input)  useSOC1=SOC2  useSOC2=SOC2_SOC3  SOCAcquisitionWindow=7  SOCTriggerSource=ePWM2_ADCSOCA  SOCInterruptTrigger=No ADCINT  Ts=-1  dType=double  postInterrupt=off  interruptSel=ADCINT1  ADCINTContinuous=off  endma=off  chdma=1  conv1=ADCINB1  conv2=ADCINA0 and ADCINB0  conv1_Type4=ADCIN0  conv2_Type4=ADCIN0 and ADCIN1
      settings: LibrarySourceBlock=c2806xlib/ADC
  Vmid1 : c2802xlib/ADC  Commented=on  blkParamProc=C2000  ADCModule=1  samplingMode=Single sample mode  ADCResolution=12-bit (Single-ended input)  useSOC1=SOC3  useSOC2=SOC0_SOC1  SOCAcquisitionWindow=10  SOCTriggerSource=ePWM2_ADCSOCA  SOCInterruptTrigger=No ADCINT  Ts=-1  dType=double  postInterrupt=off  interruptSel=ADCINT1  ADCINTContinuous=on  endma=off  chdma=1  conv1=ADCINA4  conv2=ADCINA0 and ADCINB0  conv1_Type4=ADCIN0  conv2_Type4=ADCIN0 and ADCIN1
      settings: LibrarySourceBlock=c2806xlib/ADC
  Vmid2 : c2802xlib/ADC  blkParamProc=C2000  ADCModule=1  samplingMode=Single sample mode  ADCResolution=12-bit (Single-ended input)  useSOC1=SOC3  useSOC2=SOC0_SOC1  SOCAcquisitionWindow=7  SOCTriggerSource=ePWM2_ADCSOCA  SOCInterruptTrigger=No ADCINT  Ts=-1  dType=double  postInterrupt=off  interruptSel=ADCINT1  ADCINTContinuous=on  endma=off  chdma=1  conv1=ADCINA4  conv2=ADCINA0 and ADCINB0  conv1_Type4=ADCIN0  conv2_Type4=ADCIN0 and ADCIN1
      settings: LibrarySourceBlock=c2806xlib/ADC
  wires:
  Vin2/1 -> Data Store Write13/1
  Inductor current2/1 -> Data Store Write9/1
  Vin5/1 -> Data Store Write7/1
  Inductor current7/1 -> Data Store Write3/1
  Vin7/1 -> Data Store Write17/1
  Inductor current5/1 -> Data Store Write6/1
  Vbulk2/1 -> Data Store Write18/1
  Inductor current6/1 -> Data Store Write4/1
  Vmid2/1 -> Data Store Write16/1
  Vin6/1 -> Data Store Write5/1
  Inductor current1/1 -> Data Store Write8/1
  Inductor current4/1 -> Data Store Write1/1
  Inductor current3/1 -> Data Store Write2/1
  Vbulk1/1 -> Data Store Write12/1
  Vin3/1 -> Data Store Write19/1
  Vin4/1 -> Data Store Write11/1
  Inductor current10/1 -> Data Store Write14/1
  Vmid1/1 -> Data Store Write10/1
  Vin1/1 -> Data Store Write21/1
  Inductor current8/1 -> Data Store Write20/1
  Inductor current9/1 -> Data Store Write15/1
